simulink model "EL"  (R2023a)
settings: Solver=VariableStepAuto  StartTime=0.0  StopTime=0.1  RelTol=1e-3
undefined symbols (not defined in the file): Ion, Lithium
libraries: spsParallelRLCBranchLib x4, spsVoltageMeasurementLib x2, spsBatteryLib x1, spsControlledCurrentSourceLib x1, spsControlledVoltageSourceLib x1, spsCurrentMeasurementLib x1, fuzblock x1, spspowerguiLib x1
settings Model: DataTypeOverride=Off  Creator=pc180  LastModifiedBy=pc180
settings OptimizationCC: DefaultUnderspecifiedDataType=single
settings SFSimCC: SimCustomHeaderCode="#include \"pid.h\""  SimUserSources=pid_test.c  CustomCodeUndefinedFunction=ThrowError  CustomCodeGlobalsAsFunctionIO=on

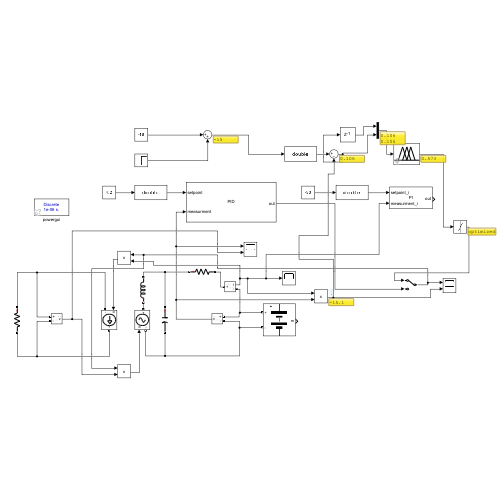
[thumbnail: Simulink's stored preview of the top-level diagram]
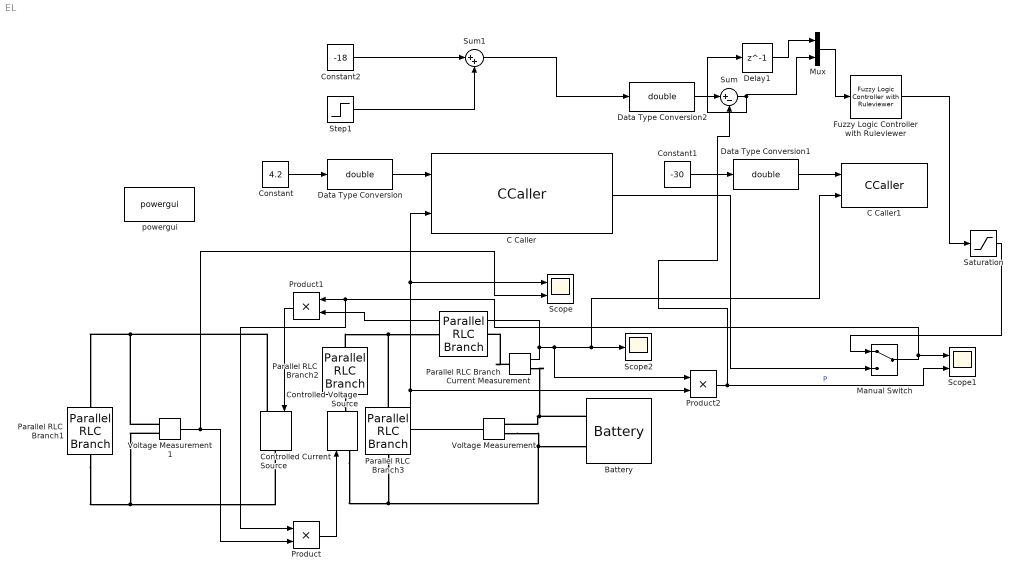
== system EL ==
  Battery : spsBatteryLib/Battery  BatType=Lithium-Ion  ShowTempParam=off  ThermalPreset=no  ShowAgeParam=off  NomV=4.2  NomQ=3.25  SOC=50  Batt_Tr=30  PresetModel=on  MaxQ=3.25  MinV=3.15  FullV=4.8887  Dis_rate=1.413  R=0.012923  Normal_OP=2.9391  expZone="[4.5376     0.15967]"  current=[6.5 13 32.5]  Units=Time  Tci=20  NomT=20  T2=-30  MaxQ2=4.8  FullV2=7.1  Normal_OP2=5.655  expZone2="[6.58           1]"  Rca=0.6  ti=2000  Dp=0  Neq0=0  Tsim=1e6  Ta1=25  Qeol=5.4*0.9  Reol=0.013333*1.2  Char_age=[2.3478, 3]  Dis_age=[2.3478, 10]  N1=1500  N2=10500  N3=1000  N4=1400  Ta2=45  N5=950
  C Caller : CCaller  FunctionName=PID  PortSpecificationStruct="%)30     .    B 4   8    (     @         %    \"     ,    !     0         %  0 \"0    $    _    07)G3F%M90  4&]R=$YA;64 4V-O<&4     26YD97@     5'EP90      4VEZ90      27-';&]B86P   X    P    !@    @    $          4    (     0    ,    !         !   P!O=70 #@   #     &    \"     0         !0    @    !     P    $         $  # &]U=  .    .     8    (    !          %    \"     $    &     0         0    !@   $]U='!U=   #@   #@    &    \"     8         !0    @    !     0    $         \"0    @               X    X    !@    @    $          4    (     0    8    !         !     &    9&]U8FQE   .    ,     8    (    !          %    \"     $    !     0         0  $ ,0    X    P    !@    @    ) @        4    (     0    $    !          (  0      #@   #@    &    \"     0         !0    @    !    \"     $         $     @   !S971P;VEN= X    X    !@    @    $          4    (     0    @    !         !     (    <V5T<&]I;G0.    .     8    (    !          %    \"     $    %     0         0    !0   $EN<'5T    #@   #@    &    \"     8         !0    @    !     0    $         \"0    @               X    X    !@    @    $          4    (     0    8    !         !     &    9&]U8FQE   .    ,     8    (    !          %    \"     $    !     0         0  $ ,0    X    P    !@    @    ) @        4    (     0    $    !          (  0      #@   $     &    \"     0         !0    @    !    \"@    $         $     H   !M96%S=7)M96YT        #@   $     &    \"     0         !0    @    !    \"@    $         $     H   !M96%S=7)M96YT        #@   #@    &    \"     0         !0    @    !    !0    $         $     4   !);G!U=     X    X    !@    @    &          4    (     0    $    !          D    (            \\#\\.    .     8    (    !          %    \"     $    &     0         0    !@   &1O=6)L90  #@   #     &    \"     0         !0    @    !     0    $         $  ! #$    .    ,     8    (    \"0(        %    \"     $    !     0         \"  $"
  C Caller1 : CCaller  FunctionName=PI  PortSpecificationStruct="%)30     .    F 4   8    (     @         %    \"     ,    !     0         %  0 \"0    $    _    07)G3F%M90  4&]R=$YA;64 4V-O<&4     26YD97@     5'EP90      4VEZ90      27-';&]B86P   X    P    !@    @    $          4    (     0    ,    !         !   P!O=70 #@   #     &    \"     0         !0    @    !     P    $         $  # &]U=  .    .     8    (    !          %    \"     $    &     0         0    !@   $]U='!U=   #@   #@    &    \"     8         !0    @    !     0    $         \"0    @               X    X    !@    @    $          4    (     0    8    !         !     &    9&]U8FQE   .    ,     8    (    !          %    \"     $    !     0         0  $ ,0    X    P    !@    @    ) @        4    (     0    $    !          (  0      #@   $     &    \"     0         !0    @    !    \"@    $         $     H   !S971P;VEN=%]I        #@   $     &    \"     0         !0    @    !    \"@    $         $     H   !S971P;VEN=%]I        #@   #@    &    \"     0         !0    @    !    !0    $         $     4   !);G!U=     X    X    !@    @    &          4    (     0    $    !          D    (               .    .     8    (    !          %    \"     $    &     0         0    !@   &1O=6)L90  #@   #     &    \"     0         !0    @    !     0    $         $  ! #$    .    ,     8    (    \"0(        %    \"     $    !     0         \"  $       X   !     !@    @    $          4    (     0    P    !         !     ,    ;65A<W5R;65N=%]I      X   !     !@    @    $          4    (     0    P    !         !     ,    ;65A<W5R;65N=%]I      X    X    !@    @    $          4    (     0    4    !         !     %    26YP=70    .    .     8    (    !@         %    \"     $    !     0         )    \"            / _#@   #@    &    \"     0         !0    @    !    !@    $         $     8   !D;W5B;&4   X    P    !@    @    $          4    (     0    $    !         !   0 Q    #@   #     &    \"     D\"        !0    @    !     0    $          @ !"
  Constant : Constant  Value=4.2  OutDataTypeStr=single  LockScale=on
  Constant1 : Constant  Value=-30  OutDataTypeStr=single  LockScale=on
  Constant2 : Constant  Value=-18  OutDataTypeStr=single  LockScale=on
  Controlled Current Source : spsControlledCurrentSourceLib/Controlled Current Source  Initialize=on  Source_Type=AC  Amplitude=0  Phase=0  Frequency=0  Measurements=None
  Controlled Voltage Source : spsControlledVoltageSourceLib/Controlled Voltage Source  Initialize=on  Source_Type=DC  Amplitude=0  Phase=0  Frequency=0  Measurements=None
  Current Measurement : spsCurrentMeasurementLib/Current Measurement  PhasorSimulation=off  OutputType=Complex  PSBequivalent=0
  Data Type Conversion : DataTypeConversion  OutDataTypeStr=double  SaturateOnIntegerOverflow=off  RndMeth=Floor
  Data Type Conversion1 : DataTypeConversion  OutDataTypeStr=double  SaturateOnIntegerOverflow=off  RndMeth=Floor
  Data Type Conversion2 : DataTypeConversion  OutDataTypeStr=double  SaturateOnIntegerOverflow=off  RndMeth=Floor
  Delay1 : Delay  DelayLength=1  InitialCondition=0
  Fuzzy Logic Controller with Ruleviewer : fuzblock/Fuzzy Logic  Controller  with Ruleviewer  fismatrix=fis_power  Ts=0.0000167
  Manual Switch : ManualSwitch
  Mux : Mux  Inputs=2
  Parallel RLC Branch : spsParallelRLCBranchLib/Parallel RLC Branch  LConnTagsString=a  RConnTagsString=__new0  BranchType=R  Resistance=1  Inductance=1e-3  SetiL0=off  InitialCurrent=0  Capacitance=1e-6  Setx0=off  InitialVoltage=0  Measurements=None
  Parallel RLC Branch1 : spsParallelRLCBranchLib/Parallel RLC Branch  LConnTagsString=a  RConnTagsString=__new0  BranchType=R  Resistance=1  Inductance=1e-3  SetiL0=off  InitialCurrent=0  Capacitance=1e-6  Setx0=off  InitialVoltage=0  Measurements=None
  Parallel RLC Branch2 : spsParallelRLCBranchLib/Parallel RLC Branch  LConnTagsString=a  RConnTagsString=__new0  BranchType=L  Resistance=1  Inductance=470e-6  SetiL0=off  InitialCurrent=0  Capacitance=1e-6  Setx0=off  InitialVoltage=0  Measurements=None
  Parallel RLC Branch3 : spsParallelRLCBranchLib/Parallel RLC Branch  LConnTagsString=a  RConnTagsString=__new0  BranchType=C  Resistance=1  Inductance=1e-3  SetiL0=off  InitialCurrent=0  Capacitance=470e-6  Setx0=off  InitialVoltage=0  Measurements=None
  Product : Product
  Product1 : Product
  Product2 : Product
  Saturation : Saturate  UpperLimit=1  LowerLimit=0
  Scope : Scope  NumInputPorts=2
  Scope1 : Scope  NumInputPorts=2
  Scope2 : Scope
  Step1 : Step  Time=50e-3  After=3  SampleTime=0
  Sum : Sum  Inputs=|+-
  Sum1 : Sum  Inputs=|++
  Voltage Measurement : spsVoltageMeasurementLib/Voltage Measurement  PhasorSimulation=off  OutputType=Complex  PSBequivalent=0
  Voltage Measurement1 : spsVoltageMeasurementLib/Voltage Measurement  PhasorSimulation=off  OutputType=Complex  PSBequivalent=0
  powergui : spspowerguiLib/powergui  Priority=1  SimulationMode=Discrete  SampleTime=1e-06  frequency=60  Iterations=50  frequencyindice=0  Pbase=100e6  ErrMax=1e-4  UnitsV=kV  UnitsW=MW  buscounter=0  FunctionMessages=off  echomessages=off  EnableUseOfTLC=off  CurrentSourceSwitches=off  DisableSnubberDevices=off  DisableRonSwitches=off  DisableVfSwitches=off  DisplayEquations=off  AutomaticDiscreteSolvers=off  SolverType=Tustin/Backward Euler (TBE)  Interpol=off  ExternalGateDelay=off  methode=off  Ts=100  x0status=blocks  SPID=on  SwTol=0  HookPort=off  NonlinearTolerance=1e-4  nMaxIteration=100  ContinueOnMaxIteration=off  RestoreLinks=warning  ResistiveCurrentMeasurement=off  Frange=[0:2:500]  Ylog=off  Xlog=on  ShowGrid=off  save=off  variable=ZData  structure=0  ZoomFFT=off  StartTime=0.0  cycles=1  DisplayStyle=1  fundamental=60  FreqAxis=off  MaxFrequency=1000  frequencyindicesteady=1  RmsSteady=1  display=off
  wires:
  Voltage Measurement/1 -> Product2/2, C Caller/2, Scope/1
  Constant/1 -> Data Type Conversion/1
  Data Type Conversion/1 -> C Caller/1
  Voltage Measurement1/1 -> Scope/2, Product/2
  Product/1 -> Controlled Voltage Source/1
  Product1/1 -> Controlled Current Source/1
  Current Measurement/1 -> Product2/1, C Caller1/2, Scope2/1, Product1/2
  Data Type Conversion1/1 -> C Caller1/1
  Constant1/1 -> Data Type Conversion1/1
  Manual Switch/1 -> Scope1/1, Product/1, Product1/1
  C Caller/1 -> Manual Switch/2
  Product2/1 -> Sum/2, Scope1/2  "P"
  Data Type Conversion2/1 -> Sum/1
  Delay1/1 -> Mux/1
  Sum/1 -> Delay1/1, Mux/2
  Mux/1 -> Fuzzy Logic Controller with Ruleviewer/1
  Fuzzy Logic Controller with Ruleviewer/1 -> Saturation/1
  Saturation/1 -> Manual Switch/1
  Sum1/1 -> Data Type Conversion2/1
  Constant2/1 -> Sum1/1
  Step1/1 -> Sum1/2
  connections:
  Battery/LConn1 -- Current Measurement/RConn1 -- Voltage Measurement/LConn1
  Controlled Voltage Source/LConn1 -- Parallel RLC Branch3/RConn1 -- Voltage Measurement/LConn2 -- Battery/LConn2
  Controlled Current Source/LConn1 -- Voltage Measurement1/LConn1 -- Parallel RLC Branch1/LConn1
  Parallel RLC Branch1/RConn1 -- Voltage Measurement1/LConn2 -- Controlled Current Source/RConn1
  Current Measurement/LConn1 -- Parallel RLC Branch/RConn1
  Parallel RLC Branch2/LConn1 -- Controlled Voltage Source/RConn1
  Parallel RLC Branch2/RConn1 -- Parallel RLC Branch3/LConn1 -- Parallel RLC Branch/LConn1
